simulink model "Corrected_STModel_with_IMM"  (R2019b)
settings: Solver=FixedStepDiscrete  StartTime=0.0  StopTime=6  FixedStep=Ts  RelTol=1e-3  EnableMultiTasking=on
PreLoadFcn:
  | if exist('tl_preloadfcn','file'), tl_preloadfcn(gcs,403); end
PostLoadFcn:
  | if exist('tl_postloadfcn','file'), tl_postloadfcn(gcs,403); end
InitFcn:
  | if exist('tlds_init','file'), tlds_init(gcs); end
StartFcn:
  | if exist('tlds_start','file'), tlds_start(gcs); end
StopFcn:
  | if exist('tlds_stop','file'), tlds_stop(gcs); end
values from neighbouring files (symbols this model uses):
  Bx_ash_f = 11.7    [correctedST_with_behavior_data.m]
  Bx_ash_r = 11.1    [correctedST_with_behavior_data.m]
  Bx_snow_f = 10.2    [correctedST_with_behavior_data.m]
  Bx_snow_r = 9.71    [correctedST_with_behavior_data.m]
  Bx_wash_f = 12    [correctedST_with_behavior_data.m]
  Bx_wash_r = 11.5    [correctedST_with_behavior_data.m]
  By_ash_f = 8.86    [correctedST_with_behavior_data.m]
  By_ash_r = 9.30    (= 9.3)    [correctedST_with_behavior_data.m]
  By_snow_f = 19.1    [correctedST_with_behavior_data.m]
  By_snow_r = 20.0    (= 20)    [correctedST_with_behavior_data.m]
  By_wash_f = 10.7    [correctedST_with_behavior_data.m]
  By_wash_r = 11.3    [correctedST_with_behavior_data.m]
  Cx_ash_f = 1.69    [correctedST_with_behavior_data.m]
  Cx_ash_r = 1.69    [correctedST_with_behavior_data.m]
  Cx_snow_f = 1.96    [correctedST_with_behavior_data.m]
  Cx_snow_r = 1.96    [correctedST_with_behavior_data.m]
  Cx_wash_f = 1.80    (= 1.8)    [correctedST_with_behavior_data.m]
  Cx_wash_r = 1.80    (= 1.8)    [correctedST_with_behavior_data.m]
  Cy_ash_f = 1.19    [correctedST_with_behavior_data.m]
  Cy_ash_r = 1.19    [correctedST_with_behavior_data.m]
  Cy_snow_f = 0.550    (= 0.55)    [correctedST_with_behavior_data.m]
  Cy_snow_r = 0.550    (= 0.55)    [correctedST_with_behavior_data.m]
  Cy_wash_f = 1.07    [correctedST_with_behavior_data.m]
  Cy_wash_r = 1.07    [correctedST_with_behavior_data.m]
  Ex_ash_f = 0.377    [correctedST_with_behavior_data.m]
  Ex_ash_r = 0.362    [correctedST_with_behavior_data.m]
  Ex_snow_f = 0.651    [correctedST_with_behavior_data.m]
  Ex_snow_r = 0.624    [correctedST_with_behavior_data.m]
  Ex_wash_f = 0.313    [correctedST_with_behavior_data.m]
  Ex_wash_r = 0.300    (= 0.3)    [correctedST_with_behavior_data.m]
  Ey_ash_f = -1.21    [correctedST_with_behavior_data.m]
  Ey_ash_r = -1.11    [correctedST_with_behavior_data.m]
  Ey_snow_f = -2.1    [correctedST_with_behavior_data.m]
  Ey_snow_r = -1.93    [correctedST_with_behavior_data.m]
  Ey_wash_f = -2.14    [correctedST_with_behavior_data.m]
  Ey_wash_r = -1.97    [correctedST_with_behavior_data.m]
  g = 9.81    [correctedST_with_behavior_data.m]
  Iw = 4    [correctedST_with_behavior_data.m]
  Iz = 2873    [correctedST_with_behavior_data.m]
  l = l_f+l_r    (= 2.68)    [correctedST_with_behavior_data.m]
  l_f = 1.1    [correctedST_with_behavior_data.m]
  l_r = 1.58    [correctedST_with_behavior_data.m]
  m = 1573    [correctedST_with_behavior_data.m]
  mu_x_ash_f = 1.20    (= 1.2)    [correctedST_with_behavior_data.m]
  mu_x_ash_r = 1.20    (= 1.2)    [correctedST_with_behavior_data.m]
  mu_x_snow_f = 0.407    [correctedST_with_behavior_data.m]
  mu_x_snow_r = 0.409    [correctedST_with_behavior_data.m]
  mu_x_wash_f = 1.06    [correctedST_with_behavior_data.m]
  mu_x_wash_r = 1.07    [correctedST_with_behavior_data.m]
  mu_y_ash_f = 0.935    [correctedST_with_behavior_data.m]
  mu_y_ash_r = 0.961    [correctedST_with_behavior_data.m]
  mu_y_snow_f = 0.383    [correctedST_with_behavior_data.m]
  mu_y_snow_r = 0.394    [correctedST_with_behavior_data.m]
  mu_y_wash_f = 0.885    [correctedST_with_behavior_data.m]
  mu_y_wash_r = 0.911    [correctedST_with_behavior_data.m]
  omega_f0 = Vx0/Rw    (= 33.3333333333)    [correctedST_with_behavior_data.m]
  omega_r0 = Vx0/Rw    (= 33.3333333333)    [correctedST_with_behavior_data.m]
  P_init = 0.0025    [correctedST_with_behavior_data.m]
  psi0 = 0    [correctedST_with_behavior_data.m]
  psi_dot0 = 0    [correctedST_with_behavior_data.m]
  Px0 = 0    [correctedST_with_behavior_data.m]
  Py0 = 0    [correctedST_with_behavior_data.m]
  Re = 0.3    [correctedST_with_behavior_data.m]
  road = 1    [correctedST_with_behavior_data.m]
  Rw = 0.3    [correctedST_with_behavior_data.m]
  Ts = 0.001    [correctedST_with_behavior_data.m]
  Ts_bp = 0.01    [correctedST_with_behavior_data.m]
  Tsmall = 0.001    [correctedST_with_behavior_data.m]
  vx = 10    [correctedST_with_behavior_data.m]
  Vx0 = 10    [correctedST_with_behavior_data.m]
  vy = 0    [correctedST_with_behavior_data.m]
  Vy0 = 0    [correctedST_with_behavior_data.m]
  x = 0    [correctedST_with_behavior_data.m]
  y = 0    [correctedST_with_behavior_data.m]
undefined symbols (not defined in the file or in its folder): DLCTest
libraries: simulink x2
PreSaveFcn:
  | if exist('tl_presavefcn','file'), tl_presavefcn(gcs); end
CloseFcn:
  | if exist('tl_closefcn','file'), tl_closefcn(gcs); end
settings Model: TLRevision=403  ExtModeTrigDuration=10000  Creator=srivats  LastModifiedBy=jasprit
settings SolverCC: PositivePriorityOrder=on  AutoInsertRateTranBlk=on
settings DataIOCC: ReturnWorkspaceOutputs=off
settings DebuggingCC: ArithmeticOperatorsInVariantConditions=warning
settings SFSimCC: SimUseLocalCustomCode=off  CustomCodeUndefinedFunction=UseInterfaceOnly
settings RTWCC: Description=QUARC Win64 Target  SystemTargetFile=quarc_win64.tlc  TemplateMakefile=quarc_default_tmf  RTWUseLocalCustomCode=off
settings STFCustomTargetCC: TargetPreCompLibLocation=C:\PROGRA~3\QUARC\lib\2018a\win64\release  TargetLangStandard=C99 (ISO)  ConcurrentExecutionCompliant=on  GRTInterface=on  SystemTargetFile=quarc_win64.tlc
settings GRTTargetCC: TargetPreCompLibLocation=C:\PROGRA~3\QUARC\lib\2018a\win64\release  ParMdlRefBuildCompliant=off  CompOptLevelCompliant=off  CombineOutputUpdateFcns=off  MatFileLogging=off  CPPClassGenCompliant=off  GRTInterface=on  UseToolchainInfoCompliant=off  ExtMode=on  ExtModeMexFile=quarc_comm

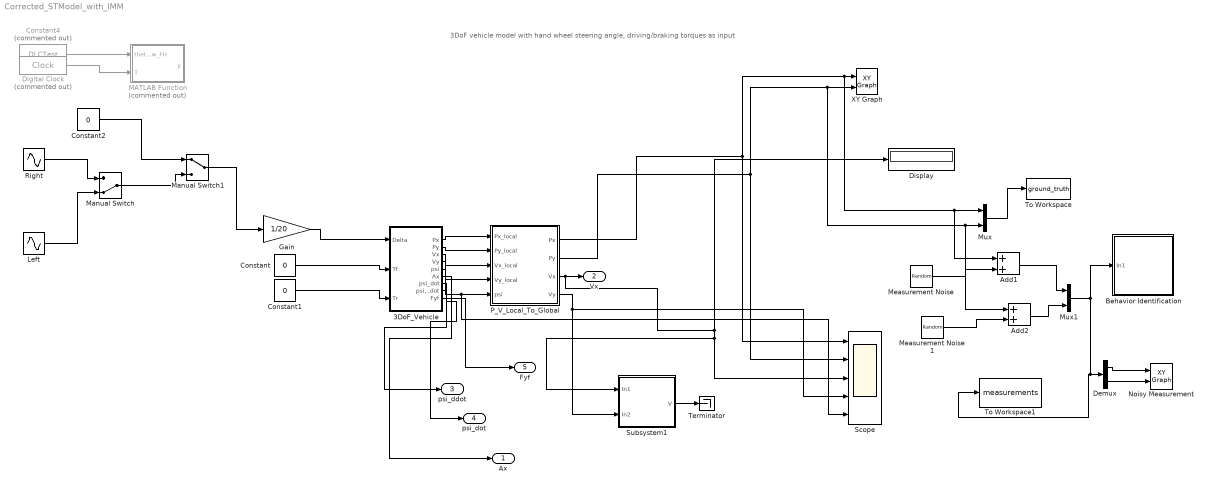
== system Corrected_STModel_with_IMM ==
  note: 3DoF vehicle model with hand wheel steering angle, driving/braking torques as input
  3DoF_Vehicle : Subsystem
  Add1 : Sum
  Add2 : Sum
  Behavior Identification : Subsystem
  Constant : Constant  Value=0
  Constant1 : Constant  Value=0
  Constant2 : Constant  Value=0
  Constant4 : Constant  Commented=on  Value=DLCTest
  Demux : Demux  Outputs=2
  Digital Clock : DigitalClock  Commented=on  SampleTime=0.001
  Display : Display
  Gain : Gain  Gain=1/20
  Left : Sin  Amplitude=0.105  Frequency=2*pi/10  SampleTime=0
  MATLAB Function : MATLAB Function  Commented=on  TreatAsAtomicUnit=on
  Manual Switch : ManualSwitch  CurrentSetting=0
  Manual Switch1 : ManualSwitch
  "Measurement Noise " : RandomNumber  Variance=0.0025
  Measurement Noise 1 : RandomNumber  Variance=0.0025
  Mux : Mux  Inputs=2
  Mux1 : Mux  Inputs=2
  Noisy Measurement : simulink/Sinks/XY Graph  xmin=-10  xmax=100  ymin=-5  ymax=5  st=-1
  P_V_Local_To_Global : Subsystem
  Right : Sin  Amplitude=0.105  Frequency=2*pi/10  Phase=-pi  SampleTime=0
  Scope : Scope  NumInputPorts=5
  Subsystem1 : Subsystem
  Terminator : Terminator
  To Workspace : ToWorkspace  VariableName=ground_truth  SaveFormat=Timeseries  SampleTime=Ts_bp
  To Workspace1 : ToWorkspace  VariableName=measurements  SaveFormat=Timeseries  SampleTime=Ts_bp
  XY Graph : simulink/Sinks/XY Graph  xmin=0  xmax=75  ymin=-4  ymax=4  st=-1
  Ax : Outport  VectorParamsAs1DForOutWhenUnconnected=off
  Vx : Outport  Port=2  VectorParamsAs1DForOutWhenUnconnected=off
  psi_ddot : Outport  Port=3  VectorParamsAs1DForOutWhenUnconnected=off
  psi_dot : Outport  Port=4  VectorParamsAs1DForOutWhenUnconnected=off
  Fyf : Outport  Port=5  VectorParamsAs1DForOutWhenUnconnected=off
  wires:
  P_V_Local_To_Global/4(Vy) -> Scope/4, Subsystem1/2(In2)
  3DoF_Vehicle/5(psi) -> Scope/5, P_V_Local_To_Global/5(psi)
  P_V_Local_To_Global/3(Vx) -> Display/1, Subsystem1/1(In1), Scope/3, Vx/1
  Subsystem1/1(V) -> Terminator/1
  Constant1/1 -> 3DoF_Vehicle/3(Tr)
  3DoF_Vehicle/4(Vy) -> P_V_Local_To_Global/4(Vy_local)
  Constant/1 -> 3DoF_Vehicle/2(Tf)
  3DoF_Vehicle/2(Py) -> P_V_Local_To_Global/2(Py_local)
  3DoF_Vehicle/3(Vx) -> P_V_Local_To_Global/3(Vx_local)
  3DoF_Vehicle/1(Px) -> P_V_Local_To_Global/1(Px_local)
  3DoF_Vehicle/6(Ax) -> Ax/1
  3DoF_Vehicle/8(psi_ddot) -> psi_ddot/1
  3DoF_Vehicle/7(psi_dot) -> psi_dot/1
  3DoF_Vehicle/9(Fyf) -> Fyf/1
  Gain/1 -> 3DoF_Vehicle/1(Delta)
  Constant4/1 -> MATLAB Function/1(theta_sw_FH)
  Digital Clock/1 -> MATLAB Function/2(T)
  Manual Switch/1 -> Manual Switch1/2
  Left/1 -> Manual Switch/2
  Mux/1 -> To Workspace/1
  P_V_Local_To_Global/2(Py) -> Add2/1, Mux/2, XY Graph/2, Scope/2
  P_V_Local_To_Global/1(Px) -> Add1/1, Mux/1, XY Graph/1, Scope/1
  Add1/1 -> Mux1/1
  Demux/1 -> Noisy Measurement/1
  Demux/2 -> Noisy Measurement/2
  Right/1 -> Manual Switch/1
  Constant2/1 -> Manual Switch1/1
  Manual Switch1/1 -> Gain/1
  "Measurement Noise "/1 -> Add1/2
  Measurement Noise 1/1 -> Add2/2
  Add2/1 -> Mux1/2
  Mux1/1 -> Behavior Identification/1(In1), To Workspace1/1, Demux/1

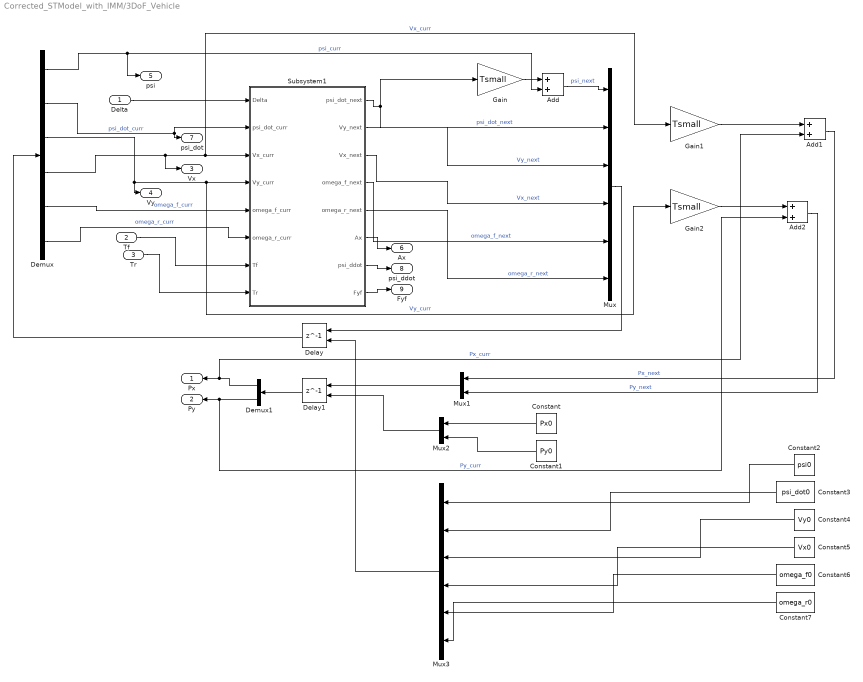
== system Corrected_STModel_with_IMM/3DoF_Vehicle ==
  Delta : Inport
  Tf : Inport  Port=2
  Tr : Inport  Port=3
  Add : Sum
  Add1 : Sum
  Add2 : Sum
  Constant : Constant  Value=Px0
  Constant1 : Constant  Value=Py0
  Constant2 : Constant  Value=psi0
  Constant3 : Constant  Value=psi_dot0
  Constant4 : Constant  Value=Vy0
  Constant5 : Constant  Value=Vx0
  Constant6 : Constant  Value=omega_f0
  Constant7 : Constant  Value=omega_r0
  Delay : Delay  DelayLength=1  InitialConditionSource=Input port  SampleTime=Tsmall
      settings: InputPortMap=u0,p4
  Delay1 : Delay  DelayLength=1  InitialConditionSource=Input port  SampleTime=Tsmall
      settings: InputPortMap=u0,p4
  Demux : Demux  Outputs=6
  Demux1 : Demux  Outputs=2
  Gain : Gain  Gain=Tsmall
  Gain1 : Gain  Gain=Tsmall
  Gain2 : Gain  Gain=Tsmall
  Mux : Mux  Inputs=6
  Mux1 : Mux  Inputs=2
  Mux2 : Mux  Inputs=2
  Mux3 : Mux  Inputs=6
  Subsystem1 : Subsystem
  Px : Outport  VectorParamsAs1DForOutWhenUnconnected=off
  Py : Outport  Port=2  VectorParamsAs1DForOutWhenUnconnected=off
  Vx : Outport  Port=3  VectorParamsAs1DForOutWhenUnconnected=off
  Vy : Outport  Port=4  VectorParamsAs1DForOutWhenUnconnected=off
  psi : Outport  Port=5  VectorParamsAs1DForOutWhenUnconnected=off
  Ax : Outport  Port=6  VectorParamsAs1DForOutWhenUnconnected=off
  psi_dot : Outport  Port=7  VectorParamsAs1DForOutWhenUnconnected=off
  psi_ddot : Outport  Port=8  VectorParamsAs1DForOutWhenUnconnected=off
  Fyf : Outport  Port=9  VectorParamsAs1DForOutWhenUnconnected=off
  wires:
  Demux/1 -> psi/1, Add/2  "psi_curr"
  Delay/1 -> Demux/1
  Demux/6 -> Subsystem1/6(omega_r_curr)  "omega_r_curr"
  Gain/1 -> Add/1
  Delta/1 -> Subsystem1/1(Delta)
  Subsystem1/4(omega_f_next) -> Mux/5  "omega_f_next"
  Subsystem1/1(psi_dot_next) -> Mux/2, Gain/1  "psi_dot_next"
  Add/1 -> Mux/1  "psi_next"
  Tr/1 -> Subsystem1/8(Tr)
  Tf/1 -> Subsystem1/7(Tf)
  Subsystem1/3(Vx_next) -> Mux/4  "Vx_next"
  Demux/2 -> psi_dot/1, Subsystem1/2(psi_dot_curr)  "psi_dot_curr"
  Mux/1 -> Delay/1
  Demux/4 -> Vx/1, Gain1/1, Subsystem1/3(Vx_curr)  "Vx_curr"
  Demux/3 -> Gain2/1, Subsystem1/4(Vy_curr), Vy/1  "Vy_curr"
  Demux/5 -> Subsystem1/5(omega_f_curr)  "omega_f_curr"
  Subsystem1/2(Vy_next) -> Mux/3  "Vy_next"
  Subsystem1/5(omega_r_next) -> Mux/6  "omega_r_next"
  Gain1/1 -> Add1/1
  Gain2/1 -> Add2/1
  Mux1/1 -> Delay1/1
  Add1/1 -> Mux1/1  "Px_next"
  Add2/1 -> Mux1/2  "Py_next"
  Mux2/1 -> Delay1/2
  Constant/1 -> Mux2/1
  Constant1/1 -> Mux2/2
  Delay1/1 -> Demux1/1
  Demux1/1 -> Add1/2, Px/1  "Px_curr"
  Demux1/2 -> Add2/2, Py/1  "Py_curr"
  Constant7/1 -> Mux3/6
  Constant6/1 -> Mux3/5
  Constant3/1 -> Mux3/2
  Constant5/1 -> Mux3/4
  Constant4/1 -> Mux3/3
  Constant2/1 -> Mux3/1
  Mux3/1 -> Delay/2
  Subsystem1/6(Ax) -> Ax/1
  Subsystem1/7(psi_ddot) -> psi_ddot/1
  Subsystem1/8(Fyf) -> Fyf/1

== system Corrected_STModel_with_IMM/Behavior Identification ==
  In1 : Inport  SampleTime=Ts_bp
  Constant : Constant  Value=0
  MATLAB Function3 : MATLAB Function  TreatAsAtomicUnit=on
  P_init : Constant  Value=P_init * eye(4)  SampleTime=-1
  To Workspace2 : ToWorkspace  VariableName=imm_comb_estimate  SaveFormat=Timeseries  SampleTime=-1
  combined Estimate : Scope
  estimates : Scope
  likelihoods : Scope
  prenormalized Wts : Scope
  weights : Scope
  x_init : Constant  Value=[x vx y vy]'
  wires:
  Constant/1 -> MATLAB Function3/2(u)
  MATLAB Function3/2(weights) -> weights/1
  MATLAB Function3/1(prenormalizedWts) -> prenormalized Wts/1
  MATLAB Function3/4(estimates) -> estimates/1
  x_init/1 -> MATLAB Function3/3(X)
  P_init/1 -> MATLAB Function3/4(P)
  MATLAB Function3/3(likelihood) -> likelihoods/1
  MATLAB Function3/5(comb_x) -> To Workspace2/1, combined Estimate/1
  In1/1 -> MATLAB Function3/1(y_tilde)

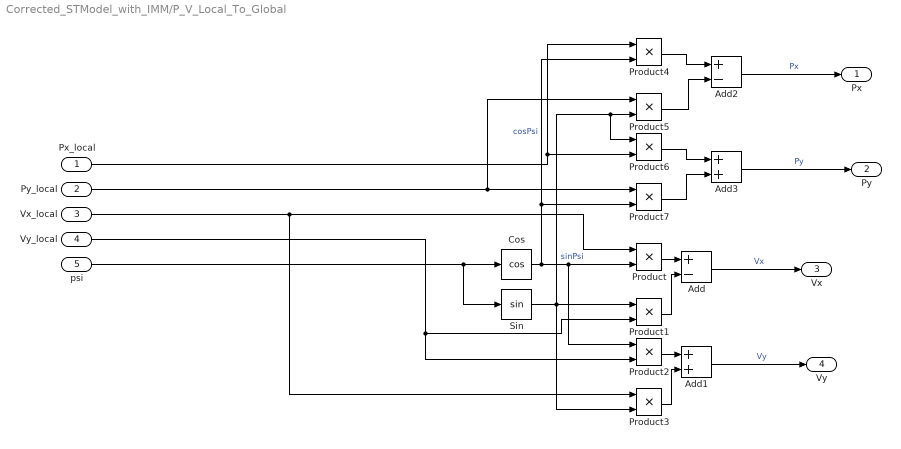
== system Corrected_STModel_with_IMM/P_V_Local_To_Global ==
  Px_local : Inport  OutDataTypeStr=double  SampleTime=Ts
  Py_local : Inport  Port=2  OutDataTypeStr=double  SampleTime=Ts
  Vx_local : Inport  Port=3  OutDataTypeStr=double  SampleTime=Ts
  Vy_local : Inport  Port=4  OutDataTypeStr=double  SampleTime=Ts
  psi : Inport  Port=5  OutDataTypeStr=double  SampleTime=Ts
  Add : Sum  Inputs=+-
  Add1 : Sum
  Add2 : Sum  Inputs=+-
  Add3 : Sum
  Cos : Trigonometry  Operator=cos
  Product{,1..7} (8 alike) : Product
  Sin : Trigonometry
  Px : Outport  OutDataTypeStr=double  SampleTime=Ts  VectorParamsAs1DForOutWhenUnconnected=off
  Py : Outport  Port=2  OutDataTypeStr=double  SampleTime=Ts  VectorParamsAs1DForOutWhenUnconnected=off
  Vx : Outport  Port=3  OutDataTypeStr=double  SampleTime=Ts  VectorParamsAs1DForOutWhenUnconnected=off
  Vy : Outport  Port=4  OutDataTypeStr=double  SampleTime=Ts  VectorParamsAs1DForOutWhenUnconnected=off
  wires:
  Px_local/1 -> Product4/1, Product6/2
  Py_local/1 -> Product7/1, Product5/1
  Vx_local/1 -> Product3/1, Product/1
  Product5/1 -> Add2/2
  Product4/1 -> Add2/1
  Add2/1 -> Px/1  "Px"
  Product7/1 -> Add3/2
  Sin/1 -> Product6/1, Product5/2, Product3/2, Product1/1  "sinPsi"
  Vy_local/1 -> Product1/2, Product2/2
  psi/1 -> Sin/1, Cos/1
  Cos/1 -> Product7/2, Product4/2, Product2/1, Product/2  "cosPsi"
  Add3/1 -> Py/1  "Py"
  Product2/1 -> Add1/1
  Product1/1 -> Add/2
  Add/1 -> Vx/1  "Vx"
  Add1/1 -> Vy/1  "Vy"
  Product6/1 -> Add3/1
  Product3/1 -> Add1/2
  Product/1 -> Add/1

== system Corrected_STModel_with_IMM/Subsystem1 ==
  In1 : Inport
  In2 : Inport  Port=2
  Add : Sum
  Sqrt : Sqrt  SaturateOnIntegerOverflow=on
  Square : Math  Operator=square  SaturateOnIntegerOverflow=on
  Square1 : Math  Operator=square  SaturateOnIntegerOverflow=on
  V : Outport  VectorParamsAs1DForOutWhenUnconnected=off
  wires:
  Square1/1 -> Add/2
  In1/1 -> Square/1
  Add/1 -> Sqrt/1
  Square/1 -> Add/1
  Sqrt/1 -> V/1  "V"
  In2/1 -> Square1/1

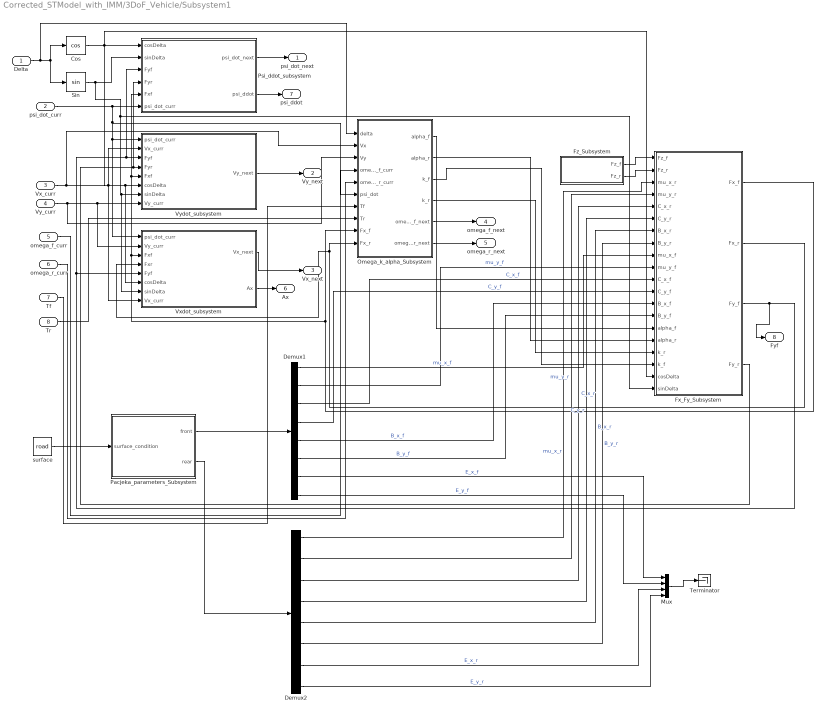
== system Corrected_STModel_with_IMM/3DoF_Vehicle/Subsystem1 ==
  Delta : Inport
  psi_dot_curr : Inport  Port=2
  Vx_curr : Inport  Port=3
  Vy_curr : Inport  Port=4
  omega_f_curr : Inport  Port=5
  omega_r_curr : Inport  Port=6
  Tf : Inport  Port=7
  Tr : Inport  Port=8
  Cos : Trigonometry  Operator=cos
  Demux1 : Demux  Outputs=8
  Demux2 : Demux  Outputs=8
  Fx_Fy_Subsystem : Subsystem
  Fz_Subsystem : Subsystem
  Mux : Mux
  Omega_k_alpha_Subsystem : Subsystem
  Pacjeka_parameters_Subsystem : Subsystem
  Psi_ddot_subsystem : Subsystem
  Sin : Trigonometry
  Terminator : Terminator
  Vxdot_subsystem : Subsystem
  Vydot_subsystem : Subsystem
  surface : Constant  Value=road
  psi_dot_next : Outport  VectorParamsAs1DForOutWhenUnconnected=off
  Vy_next : Outport  Port=2  VectorParamsAs1DForOutWhenUnconnected=off
  Vx_next : Outport  Port=3  VectorParamsAs1DForOutWhenUnconnected=off
  omega_f_next : Outport  Port=4  VectorParamsAs1DForOutWhenUnconnected=off
  omega_r_next : Outport  Port=5  VectorParamsAs1DForOutWhenUnconnected=off
  Ax : Outport  Port=6  VectorParamsAs1DForOutWhenUnconnected=off
  psi_ddot : Outport  Port=7  VectorParamsAs1DForOutWhenUnconnected=off
  Fyf : Outport  Port=8  VectorParamsAs1DForOutWhenUnconnected=off
  wires:
  Omega_k_alpha_Subsystem/4(k_r) -> Fx_Fy_Subsystem/17(k_r)
  Fx_Fy_Subsystem/2(Fx_r) -> Vxdot_subsystem/4(Fxr), Omega_k_alpha_Subsystem/10(Fx_r)
  Fx_Fy_Subsystem/1(Fx_f) -> Omega_k_alpha_Subsystem/9(Fx_f), Vxdot_subsystem/3(Fxf), Psi_ddot_subsystem/5(Fxf), Vydot_subsystem/5(Fxf)
  Omega_k_alpha_Subsystem/3(k_f) -> Fx_Fy_Subsystem/18(k_f)
  Sin/1 -> Fx_Fy_Subsystem/20(sinDelta), Vxdot_subsystem/7(sinDelta), Vydot_subsystem/7(sinDelta), Psi_ddot_subsystem/2(sinDelta)
  Vydot_subsystem/1(Vy_next) -> Vy_next/1
  Fx_Fy_Subsystem/3(Fy_f) -> Fyf/1, Psi_ddot_subsystem/3(Fyf), Vydot_subsystem/3(Fyf), Vxdot_subsystem/5(Fyf)
  psi_dot_curr/1 -> Omega_k_alpha_Subsystem/6(psi_dot), Vydot_subsystem/1(psi_dot_curr), Vxdot_subsystem/1(psi_dot_curr), Psi_ddot_subsystem/6(psi_dot_curr)
  Fx_Fy_Subsystem/4(Fy_r) -> Psi_ddot_subsystem/4(Fyr), Vydot_subsystem/4(Fyr)
  Cos/1 -> Fx_Fy_Subsystem/19(cosDelta), Vxdot_subsystem/6(cosDelta), Vydot_subsystem/6(cosDelta), Psi_ddot_subsystem/1(cosDelta)
  Tf/1 -> Omega_k_alpha_Subsystem/7(Tf)
  omega_f_curr/1 -> Omega_k_alpha_Subsystem/4(omega_f_curr)
  Vy_curr/1 -> Omega_k_alpha_Subsystem/3(Vy), Vxdot_subsystem/2(Vy_curr), Vydot_subsystem/8(Vy_curr)
  Pacjeka_parameters_Subsystem/1(front) -> Demux1/1
  Omega_k_alpha_Subsystem/6(omega_r_next) -> omega_r_next/1
  Delta/1 -> Omega_k_alpha_Subsystem/1(delta), Sin/1, Cos/1
  Vx_curr/1 -> Omega_k_alpha_Subsystem/2(Vx), Vydot_subsystem/2(Vx_curr), Vxdot_subsystem/8(Vx_curr)
  Demux1/1 -> Fx_Fy_Subsystem/9(mu_x_f)  "mu_x_f"
  Vxdot_subsystem/1(Vx_next) -> Vx_next/1
  Omega_k_alpha_Subsystem/5(omega_f_next) -> omega_f_next/1
  Demux2/4 -> Fx_Fy_Subsystem/6(C_y_r)  "C_y_r"
  Fz_Subsystem/1(Fz_f) -> Fx_Fy_Subsystem/1(Fz_f)
  Tr/1 -> Omega_k_alpha_Subsystem/8(Tr)
  omega_r_curr/1 -> Omega_k_alpha_Subsystem/5(omega_r_curr)
  surface/1 -> Pacjeka_parameters_Subsystem/1(surface_condition)
  Pacjeka_parameters_Subsystem/2(rear) -> Demux2/1
  Fz_Subsystem/2(Fz_r) -> Fx_Fy_Subsystem/2(Fz_r)
  Demux1/6 -> Fx_Fy_Subsystem/14(B_y_f)  "B_y_f"
  Demux2/6 -> Fx_Fy_Subsystem/8(B_y_r)  "B_y_r"
  Demux2/2 -> Fx_Fy_Subsystem/4(mu_y_r)  "mu_y_r"
  Demux2/5 -> Fx_Fy_Subsystem/7(B_x_r)  "B_x_r"
  Psi_ddot_subsystem/1(psi_dot_next) -> psi_dot_next/1
  Demux2/1 -> Fx_Fy_Subsystem/3(mu_x_r)  "mu_x_r"
  Demux1/3 -> Fx_Fy_Subsystem/11(C_x_f)  "C_x_f"
  Demux1/4 -> Fx_Fy_Subsystem/12(C_y_f)  "C_y_f"
  Demux1/2 -> Fx_Fy_Subsystem/10(mu_y_f)  "mu_y_f"
  Demux1/5 -> Fx_Fy_Subsystem/13(B_x_f)  "B_x_f"
  Demux2/3 -> Fx_Fy_Subsystem/5(C_x_r)  "C_x_r"
  Vxdot_subsystem/2(Ax) -> Ax/1
  Psi_ddot_subsystem/2(psi_ddot) -> psi_ddot/1
  Omega_k_alpha_Subsystem/1(alpha_f) -> Fx_Fy_Subsystem/15(alpha_f)
  Omega_k_alpha_Subsystem/2(alpha_r) -> Fx_Fy_Subsystem/16(alpha_r)
  Demux1/8 -> Mux/2  "E_y_f"
  Demux1/7 -> Mux/1  "E_x_f"
  Demux2/7 -> Mux/3  "E_x_r"
  Demux2/8 -> Mux/4  "E_y_r"
  Mux/1 -> Terminator/1

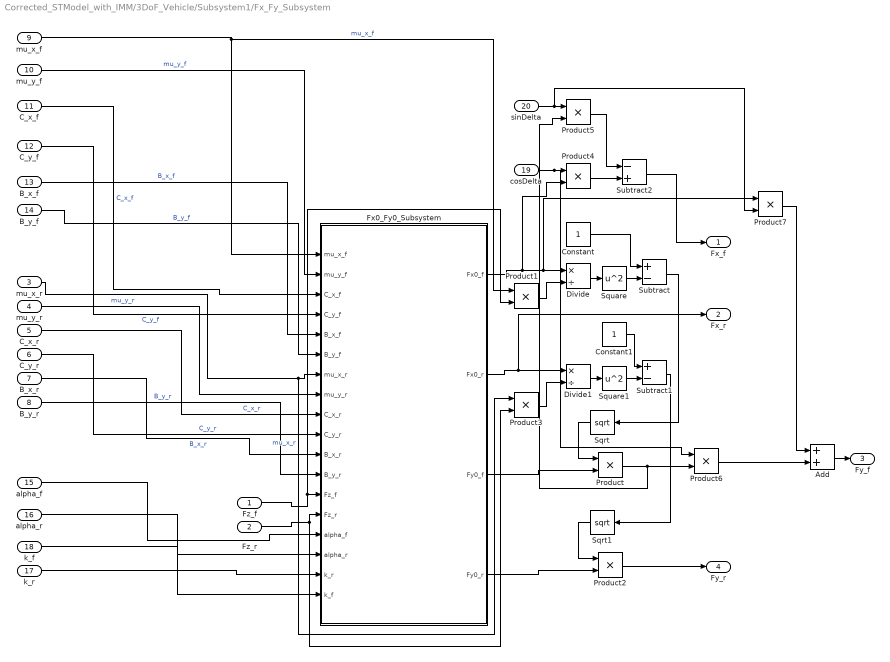
== system Corrected_STModel_with_IMM/3DoF_Vehicle/Subsystem1/Fx_Fy_Subsystem ==
  Fz_f : Inport
  Fz_r : Inport  Port=2
  mu_x_r : Inport  Port=3
  mu_y_r : Inport  Port=4
  C_x_r : Inport  Port=5
  C_y_r : Inport  Port=6
  B_x_r : Inport  Port=7
  B_y_r : Inport  Port=8
  mu_x_f : Inport  Port=9
  mu_y_f : Inport  Port=10
  C_x_f : Inport  Port=11
  C_y_f : Inport  Port=12
  B_x_f : Inport  Port=13
  B_y_f : Inport  Port=14
  alpha_f : Inport  Port=15
  alpha_r : Inport  Port=16
  k_r : Inport  Port=17
  k_f : Inport  Port=18
  cosDelta : Inport  Port=19
  sinDelta : Inport  Port=20
  Add : Sum
  Constant : Constant
  Constant1 : Constant
  Divide : Product  Inputs=*/
  Divide1 : Product  Inputs=*/
  Fx0_Fy0_Subsystem : Subsystem
  Product{,1..7} (8 alike) : Product
  Sqrt : Sqrt  SaturateOnIntegerOverflow=on
  Sqrt1 : Sqrt  SaturateOnIntegerOverflow=on
  Square : Math  Operator=square  SaturateOnIntegerOverflow=on
  Square1 : Math  Operator=square  SaturateOnIntegerOverflow=on
  Subtract : Sum  Inputs=+-
  Subtract1 : Sum  Inputs=+-
  Subtract2 : Sum  Inputs=-+
  Fx_f : Outport  VectorParamsAs1DForOutWhenUnconnected=off
  Fx_r : Outport  Port=2  VectorParamsAs1DForOutWhenUnconnected=off
  Fy_f : Outport  Port=3  VectorParamsAs1DForOutWhenUnconnected=off
  Fy_r : Outport  Port=4  VectorParamsAs1DForOutWhenUnconnected=off
  wires:
  B_x_r/1 -> Fx0_Fy0_Subsystem/11(B_x_r)  "B_x_r"
  mu_y_r/1 -> Fx0_Fy0_Subsystem/8(mu_y_r)  "mu_y_r"
  C_x_r/1 -> Fx0_Fy0_Subsystem/9(C_x_r)  "C_x_r"
  mu_x_r/1 -> Fx0_Fy0_Subsystem/7(mu_x_r), Product3/1  "mu_x_r"
  C_y_r/1 -> Fx0_Fy0_Subsystem/10(C_y_r)  "C_y_r"
  B_y_r/1 -> Fx0_Fy0_Subsystem/12(B_y_r)  "B_y_r"
  B_x_f/1 -> Fx0_Fy0_Subsystem/5(B_x_f)  "B_x_f"
  mu_y_f/1 -> Fx0_Fy0_Subsystem/2(mu_y_f)  "mu_y_f"
  C_x_f/1 -> Fx0_Fy0_Subsystem/3(C_x_f)  "C_x_f"
  mu_x_f/1 -> Product1/1, Fx0_Fy0_Subsystem/1(mu_x_f)  "mu_x_f"
  C_y_f/1 -> Fx0_Fy0_Subsystem/4(C_y_f)  "C_y_f"
  B_y_f/1 -> Fx0_Fy0_Subsystem/6(B_y_f)  "B_y_f"
  Fz_f/1 -> Product1/2, Fx0_Fy0_Subsystem/13(Fz_f)
  Fz_r/1 -> Product3/2, Fx0_Fy0_Subsystem/14(Fz_r)
  alpha_f/1 -> Fx0_Fy0_Subsystem/15(alpha_f)
  alpha_r/1 -> Fx0_Fy0_Subsystem/16(alpha_r)
  k_f/1 -> Fx0_Fy0_Subsystem/18(k_f)
  k_r/1 -> Fx0_Fy0_Subsystem/17(k_r)
  Constant/1 -> Subtract/1
  Fx0_Fy0_Subsystem/1(Fx0_f) -> Product4/2, Product7/1, Divide/1
  Product1/1 -> Divide/2
  Divide/1 -> Square/1
  Subtract/1 -> Sqrt/1
  Square/1 -> Subtract/2
  Sqrt/1 -> Product/1
  Product/1 -> Product6/2, Product5/2
  Product2/1 -> Fy_r/1
  Fx0_Fy0_Subsystem/4(Fy0_r) -> Product2/2
  Sqrt1/1 -> Product2/1
  Divide1/1 -> Square1/1
  Square1/1 -> Subtract1/2
  Product3/1 -> Divide1/2
  Fx0_Fy0_Subsystem/2(Fx0_r) -> Fx_r/1, Divide1/1
  Constant1/1 -> Subtract1/1
  Subtract1/1 -> Sqrt1/1
  cosDelta/1 -> Product6/1, Product4/1
  Product4/1 -> Subtract2/2
  sinDelta/1 -> Product7/2, Product5/1
  Fx0_Fy0_Subsystem/3(Fy0_f) -> Product/2
  Product5/1 -> Subtract2/1
  Subtract2/1 -> Fx_f/1
  Product7/1 -> Add/1
  Product6/1 -> Add/2
  Add/1 -> Fy_f/1

== system Corrected_STModel_with_IMM/3DoF_Vehicle/Subsystem1/Fz_Subsystem ==
  Constant : Constant  Value=(m*g*l_f)/l
  Constant1 : Constant  Value=(m*g*l_r)/l
  Fz_f : Outport  VectorParamsAs1DForOutWhenUnconnected=off
  Fz_r : Outport  Port=2  VectorParamsAs1DForOutWhenUnconnected=off
  wires:
  Constant/1 -> Fz_r/1
  Constant1/1 -> Fz_f/1

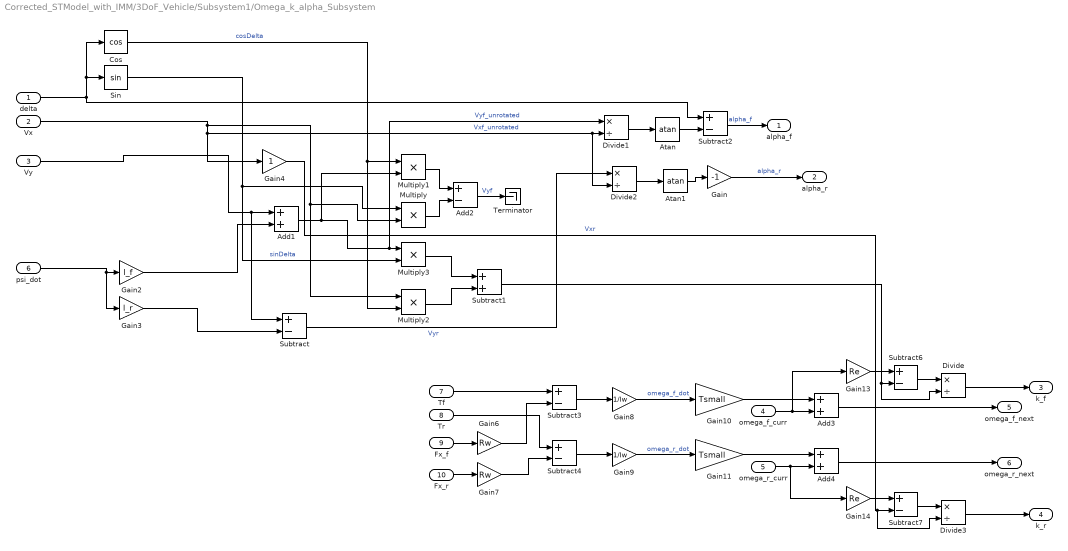
== system Corrected_STModel_with_IMM/3DoF_Vehicle/Subsystem1/Omega_k_alpha_Subsystem ==
  delta : Inport
  Vx : Inport  Port=2
  Vy : Inport  Port=3
  omega_f_curr : Inport  Port=4
  omega_r_curr : Inport  Port=5
  psi_dot : Inport  Port=6
  Tf : Inport  Port=7
  Tr : Inport  Port=8
  Fx_f : Inport  Port=9
  Fx_r : Inport  Port=10
  Add1 : Sum
  Add2 : Sum  Inputs=+-
  Add3 : Sum
  Add4 : Sum
  Atan : Trigonometry  Operator=atan
  Atan1 : Trigonometry  Operator=atan
  Cos : Trigonometry  Operator=cos
  Divide{,1..3} (4 alike) : Product  Inputs=*/
  Gain : Gain  Gain=-1
  Gain10 : Gain  Gain=Tsmall
  Gain11 : Gain  Gain=Tsmall
  Gain13 : Gain  Gain=Re
  Gain14 : Gain  Gain=Re
  Gain2 : Gain  Gain=l_f
  Gain3 : Gain  Gain=l_r
  Gain4 : Gain
  Gain6 : Gain  Gain=Rw
  Gain7 : Gain  Gain=Rw
  Gain8 : Gain  Gain=1/Iw
  Gain9 : Gain  Gain=1/Iw
  Multiply{,1..3} (4 alike) : Product
  Sin : Trigonometry
  Subtract{,2..4,6..7} (6 alike) : Sum  Inputs=+-
  Subtract1 : Sum
  Terminator : Terminator
  alpha_f : Outport  VectorParamsAs1DForOutWhenUnconnected=off
  alpha_r : Outport  Port=2  VectorParamsAs1DForOutWhenUnconnected=off
  k_f : Outport  Port=3  VectorParamsAs1DForOutWhenUnconnected=off
  k_r : Outport  Port=4  VectorParamsAs1DForOutWhenUnconnected=off
  omega_f_next : Outport  Port=5  VectorParamsAs1DForOutWhenUnconnected=off
  omega_r_next : Outport  Port=6  VectorParamsAs1DForOutWhenUnconnected=off
  wires:
  Fx_f/1 -> Gain6/1
  Fx_r/1 -> Gain7/1
  Tf/1 -> Subtract3/1
  Gain6/1 -> Subtract3/2
  Tr/1 -> Subtract4/1
  Gain7/1 -> Subtract4/2
  Subtract3/1 -> Gain8/1
  Subtract4/1 -> Gain9/1
  Gain8/1 -> Gain10/1  "omega_f_dot"
  Gain9/1 -> Gain11/1  "omega_r_dot"
  Gain10/1 -> Add3/1
  Gain11/1 -> Add4/1
  Add3/1 -> omega_f_next/1
  Add4/1 -> omega_r_next/1
  omega_f_curr/1 -> Gain13/1, Add3/2
  omega_r_curr/1 -> Gain14/1, Add4/2
  psi_dot/1 -> Gain3/1, Gain2/1
  Gain2/1 -> Add1/2
  Vy/1 -> Subtract/1, Add1/1
  Add1/1 -> Multiply1/2, Divide1/1, Multiply3/1  "Vyf_unrotated"
  Gain3/1 -> Subtract/2
  Vx/1 -> Gain4/1, Divide2/2, Divide1/2, Multiply/2, Multiply2/1  "Vxf_unrotated"
  Gain4/1 -> Divide3/2, Subtract7/2  "Vxr"
  delta/1 -> Cos/1, Sin/1, Subtract2/1
  Cos/1 -> Multiply2/2, Multiply1/1  "cosDelta"
  Multiply1/1 -> Add2/1
  Multiply/1 -> Add2/2
  Multiply3/1 -> Subtract1/1
  Multiply2/1 -> Subtract1/2
  Gain13/1 -> Subtract6/1
  Subtract6/1 -> Divide/1
  Divide/1 -> k_f/1
  Gain14/1 -> Subtract7/1
  Subtract7/1 -> Divide3/1
  Divide3/1 -> k_r/1
  Sin/1 -> Multiply/1, Multiply3/2  "sinDelta"
  Subtract1/1 -> Divide/2, Subtract6/2
  Subtract/1 -> Divide2/1  "Vyr"
  Divide1/1 -> Atan/1
  Atan/1 -> Subtract2/2
  Subtract2/1 -> alpha_f/1  "alpha_f"
  Divide2/1 -> Atan1/1
  Atan1/1 -> Gain/1
  Gain/1 -> alpha_r/1  "alpha_r"
  Add2/1 -> Terminator/1  "Vyf"

== system Corrected_STModel_with_IMM/3DoF_Vehicle/Subsystem1/Pacjeka_parameters_Subsystem ==
  surface_condition : Inport  OutDataTypeStr=double  SampleTime=Ts
  Ashphalt_condition_subsystem : Subsystem  TreatAsAtomicUnit=on
  Demux : Demux  Outputs=2
  Ice_condition_subsystem : Subsystem  TreatAsAtomicUnit=on
  Merge : Merge  Inputs=4
  Snow_condition_subsystem : Subsystem  TreatAsAtomicUnit=on
  Switch Case : SwitchCase  CaseConditions={1,2,3,4}  ShowDefaultCase=off
  WetAshphalt_condition_subsystem : Subsystem  TreatAsAtomicUnit=on
  front : Outport  OutDataTypeStr=double  SampleTime=Ts  VectorParamsAs1DForOutWhenUnconnected=off
  rear : Outport  Port=2  OutDataTypeStr=double  SampleTime=Ts  VectorParamsAs1DForOutWhenUnconnected=off
  wires:
  Demux/2 -> rear/1  "rear"
  Merge/1 -> Demux/1
  Switch Case/1 -> Ashphalt_condition_subsystem/Action
  Switch Case/3 -> Snow_condition_subsystem/Action
  Demux/1 -> front/1  "front"
  surface_condition/1 -> Switch Case/1
  Ashphalt_condition_subsystem/1(Out1) -> Merge/1
  Switch Case/2 -> WetAshphalt_condition_subsystem/Action
  WetAshphalt_condition_subsystem/1(Out1) -> Merge/2
  Snow_condition_subsystem/1(Out1) -> Merge/3
  Ice_condition_subsystem/1(Out1) -> Merge/4
  Switch Case/4 -> Ice_condition_subsystem/Action

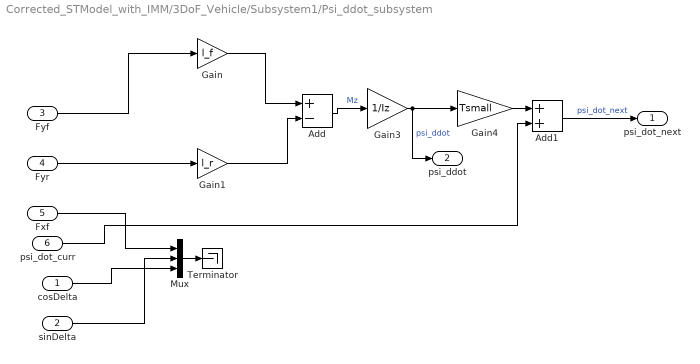
== system Corrected_STModel_with_IMM/3DoF_Vehicle/Subsystem1/Psi_ddot_subsystem ==
  cosDelta : Inport
  sinDelta : Inport  Port=2
  Fyf : Inport  Port=3
  Fyr : Inport  Port=4
  Fxf : Inport  Port=5
  psi_dot_curr : Inport  Port=6
  Add : Sum  Inputs=+-
  Add1 : Sum
  Gain : Gain  Gain=l_f
  Gain1 : Gain  Gain=l_r
  Gain3 : Gain  Gain=1/Iz
  Gain4 : Gain  Gain=Tsmall
  Mux : Mux  Inputs=3
  Terminator : Terminator
  psi_dot_next : Outport  VectorParamsAs1DForOutWhenUnconnected=off
  psi_ddot : Outport  Port=2  VectorParamsAs1DForOutWhenUnconnected=off
  wires:
  Gain/1 -> Add/1
  Gain1/1 -> Add/2
  Add/1 -> Gain3/1  "Mz"
  Gain3/1 -> psi_ddot/1, Gain4/1  "psi_ddot"
  Gain4/1 -> Add1/1
  Add1/1 -> psi_dot_next/1  "psi_dot_next"
  Fyf/1 -> Gain/1
  Fyr/1 -> Gain1/1
  psi_dot_curr/1 -> Add1/2
  cosDelta/1 -> Mux/3
  Fxf/1 -> Mux/1
  sinDelta/1 -> Mux/2
  Mux/1 -> Terminator/1

== system Corrected_STModel_with_IMM/3DoF_Vehicle/Subsystem1/Vxdot_subsystem ==
  psi_dot_curr : Inport
  Vy_curr : Inport  Port=2
  Fxf : Inport  Port=3
  Fxr : Inport  Port=4
  Fyf : Inport  Port=5
  cosDelta : Inport  Port=6
  sinDelta : Inport  Port=7
  Vx_curr : Inport  Port=8
  Add : Sum
  Fy_subsystem : Subsystem
  Gain : Gain  Gain=1/m
  Gain1 : Gain  Gain=Ts
  Multiply : Product
  Subtract : Sum
  Vx_next : Outport  VectorParamsAs1DForOutWhenUnconnected=off
  Ax : Outport  Port=2  VectorParamsAs1DForOutWhenUnconnected=off
  wires:
  sinDelta/1 -> Fy_subsystem/5(sinDelta)
  cosDelta/1 -> Fy_subsystem/4(cosDelta)
  Fyf/1 -> Fy_subsystem/3(Fxr)
  Fxr/1 -> Fy_subsystem/2(Fxf)
  Fxf/1 -> Fy_subsystem/1(Fyf)
  Fy_subsystem/1(Fx) -> Gain/1
  Gain/1 -> Subtract/2
  psi_dot_curr/1 -> Multiply/1
  Vy_curr/1 -> Multiply/2
  Multiply/1 -> Subtract/1
  Subtract/1 -> Ax/1, Gain1/1
  Gain1/1 -> Add/1
  Vx_curr/1 -> Add/2
  Add/1 -> Vx_next/1  "Vx_next"

== system Corrected_STModel_with_IMM/3DoF_Vehicle/Subsystem1/Vydot_subsystem ==
  psi_dot_curr : Inport
  Vx_curr : Inport  Port=2
  Fyf : Inport  Port=3
  Fyr : Inport  Port=4
  Fxf : Inport  Port=5
  cosDelta : Inport  Port=6
  sinDelta : Inport  Port=7
  Vy_curr : Inport  Port=8
  Add : Sum
  Fy_subsystem : Subsystem
  Gain : Gain  Gain=1/m
  Gain1 : Gain  Gain=Ts
  Multiply : Product
  Subtract : Sum  Inputs=-+
  Vy_next : Outport  VectorParamsAs1DForOutWhenUnconnected=off
  wires:
  sinDelta/1 -> Fy_subsystem/5(sinDelta)
  cosDelta/1 -> Fy_subsystem/4(cosDelta)
  Fxf/1 -> Fy_subsystem/3(Fxf)
  Fyr/1 -> Fy_subsystem/2(Fyr)
  Fyf/1 -> Fy_subsystem/1(Fyf)
  Fy_subsystem/1(Fy) -> Gain/1
  Gain/1 -> Subtract/2
  psi_dot_curr/1 -> Multiply/1
  Vx_curr/1 -> Multiply/2
  Multiply/1 -> Subtract/1
  Subtract/1 -> Gain1/1
  Gain1/1 -> Add/1
  Vy_curr/1 -> Add/2
  Add/1 -> Vy_next/1  "Vy_next"

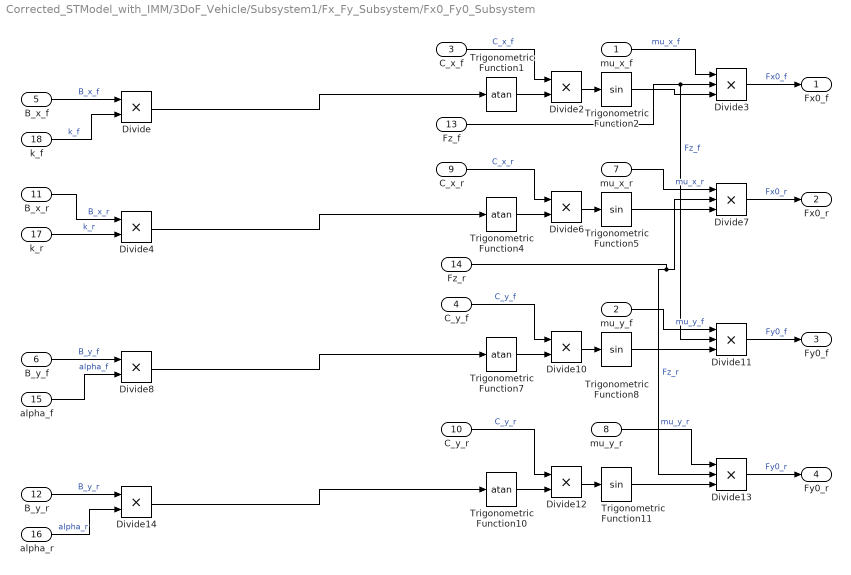
== system Corrected_STModel_with_IMM/3DoF_Vehicle/Subsystem1/Fx_Fy_Subsystem/Fx0_Fy0_Subsystem ==
  mu_x_f : Inport
  mu_y_f : Inport  Port=2
  C_x_f : Inport  Port=3
  C_y_f : Inport  Port=4
  B_x_f : Inport  Port=5
  B_y_f : Inport  Port=6
  mu_x_r : Inport  Port=7
  mu_y_r : Inport  Port=8
  C_x_r : Inport  Port=9
  C_y_r : Inport  Port=10
  B_x_r : Inport  Port=11
  B_y_r : Inport  Port=12
  Fz_f : Inport  Port=13
  Fz_r : Inport  Port=14
  alpha_f : Inport  Port=15
  alpha_r : Inport  Port=16
  k_r : Inport  Port=17
  k_f : Inport  Port=18
  Divide{,2,4,6,8,10,12,14} (8 alike) : Product  Inputs=**
  Divide{3,7,11,13} (4 alike) : Product  Inputs=***
  Trigonometric Function{1,4,7,10} (4 alike) : Trigonometry  Operator=atan
  Trigonometric Function{2,5,8,11} (4 alike) : Trigonometry
  Fx0_f : Outport  VectorParamsAs1DForOutWhenUnconnected=off
  Fx0_r : Outport  Port=2  VectorParamsAs1DForOutWhenUnconnected=off
  Fy0_f : Outport  Port=3  VectorParamsAs1DForOutWhenUnconnected=off
  Fy0_r : Outport  Port=4  VectorParamsAs1DForOutWhenUnconnected=off
  wires:
  B_x_f/1 -> Divide/1  "B_x_f"
  C_x_f/1 -> Divide2/1  "C_x_f"
  mu_x_f/1 -> Divide3/1  "mu_x_f"
  mu_y_f/1 -> Divide11/1  "mu_y_f"
  B_y_f/1 -> Divide8/1  "B_y_f"
  C_y_f/1 -> Divide10/1  "C_y_f"
  B_y_r/1 -> Divide14/1  "B_y_r"
  mu_x_r/1 -> Divide7/1  "mu_x_r"
  B_x_r/1 -> Divide4/1  "B_x_r"
  mu_y_r/1 -> Divide13/1  "mu_y_r"
  C_y_r/1 -> Divide12/1  "C_y_r"
  C_x_r/1 -> Divide6/1  "C_x_r"
  Trigonometric Function2/1 -> Divide3/3
  Divide3/1 -> Fx0_f/1  "Fx0_f"
  Trigonometric Function5/1 -> Divide7/3
  Divide4/1 -> Trigonometric Function4/1
  Divide2/1 -> Trigonometric Function2/1
  Divide/1 -> Trigonometric Function1/1
  Trigonometric Function4/1 -> Divide6/2
  Divide7/1 -> Fx0_r/1  "Fx0_r"
  Divide6/1 -> Trigonometric Function5/1
  Trigonometric Function1/1 -> Divide2/2
  alpha_f/1 -> Divide8/2  "alpha_f"
  alpha_r/1 -> Divide14/2  "alpha_r"
  k_f/1 -> Divide/2  "k_f"
  k_r/1 -> Divide4/2  "k_r"
  Trigonometric Function7/1 -> Divide10/2
  Divide10/1 -> Trigonometric Function8/1
  Fz_f/1 -> Divide11/2, Divide3/2  "Fz_f"
  Divide8/1 -> Trigonometric Function7/1
  Trigonometric Function8/1 -> Divide11/3
  Divide11/1 -> Fy0_f/1  "Fy0_f"
  Divide13/1 -> Fy0_r/1  "Fy0_r"
  Fz_r/1 -> Divide13/2, Divide7/2  "Fz_r"
  Divide14/1 -> Trigonometric Function10/1
  Trigonometric Function10/1 -> Divide12/2
  Trigonometric Function11/1 -> Divide13/3
  Divide12/1 -> Trigonometric Function11/1

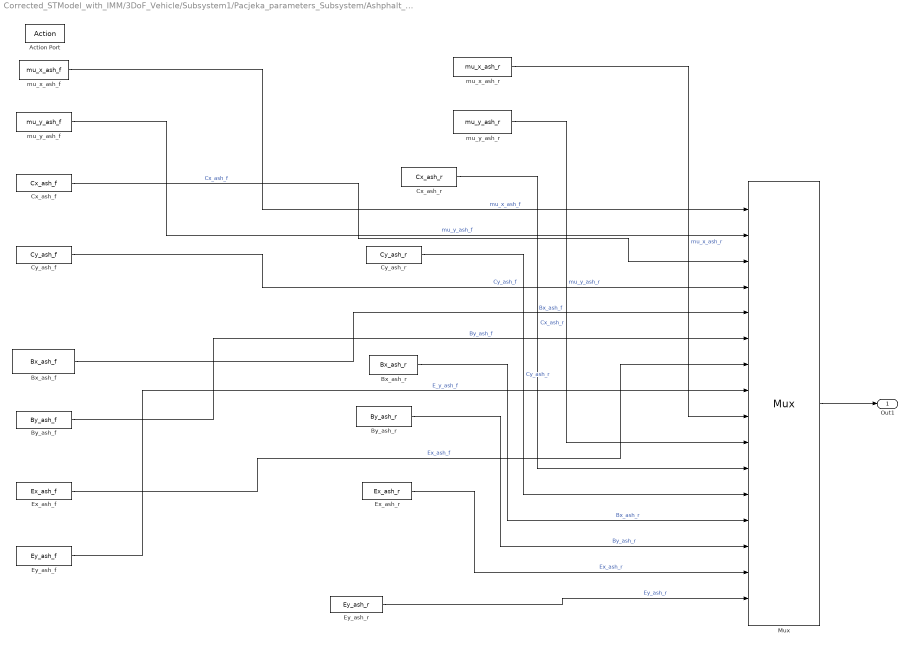
== system Corrected_STModel_with_IMM/3DoF_Vehicle/Subsystem1/Pacjeka_parameters_Subsystem/Ashphalt_condition_subsystem ==
  Action Port : ActionPort  ActionPortLabel=case [ 1 ]:
  Bx_ash_f : Constant  Value=Bx_ash_f
  Bx_ash_r : Constant  Value=Bx_ash_r
  By_ash_f : Constant  Value=By_ash_f
  By_ash_r : Constant  Value=By_ash_r
  Cx_ash_f : Constant  Value=Cx_ash_f
  Cx_ash_r : Constant  Value=Cx_ash_r
  Cy_ash_f : Constant  Value=Cy_ash_f
  Cy_ash_r : Constant  Value=Cy_ash_r
  Ex_ash_f : Constant  Value=Ex_ash_f
  Ex_ash_r : Constant  Value=Ex_ash_r
  Ey_ash_f : Constant  Value=Ey_ash_f
  Ey_ash_r : Constant  Value=Ey_ash_r
  Mux : Mux  Inputs=16
      settings: DisplayOption=signals
  mu_x_ash_f : Constant  Value=mu_x_ash_f
  mu_x_ash_r : Constant  Value=mu_x_ash_r
  mu_y_ash_f : Constant  Value=mu_y_ash_f
  mu_y_ash_r : Constant  Value=mu_y_ash_r
  Out1 : Outport  OutDataTypeStr=double  SampleTime=Ts  VectorParamsAs1DForOutWhenUnconnected=off
  wires:
  mu_x_ash_f/1 -> Mux/1  "mu_x_ash_f"
  mu_y_ash_f/1 -> Mux/2  "mu_y_ash_f"
  Cx_ash_f/1 -> Mux/3  "Cx_ash_f"
  Cy_ash_f/1 -> Mux/4  "Cy_ash_f"
  Bx_ash_f/1 -> Mux/5  "Bx_ash_f"
  By_ash_f/1 -> Mux/6  "By_ash_f"
  Ex_ash_f/1 -> Mux/7  "Ex_ash_f"
  Ey_ash_f/1 -> Mux/8  "E_y_ash_f"
  Cy_ash_r/1 -> Mux/12  "Cy_ash_r"
  Cx_ash_r/1 -> Mux/11  "Cx_ash_r"
  By_ash_r/1 -> Mux/14  "By_ash_r"
  Bx_ash_r/1 -> Mux/13  "Bx_ash_r"
  mu_y_ash_r/1 -> Mux/10  "mu_y_ash_r"
  Ex_ash_r/1 -> Mux/15  "Ex_ash_r"
  mu_x_ash_r/1 -> Mux/9  "mu_x_ash_r"
  Ey_ash_r/1 -> Mux/16  "Ey_ash_r"
  Mux/1 -> Out1/1

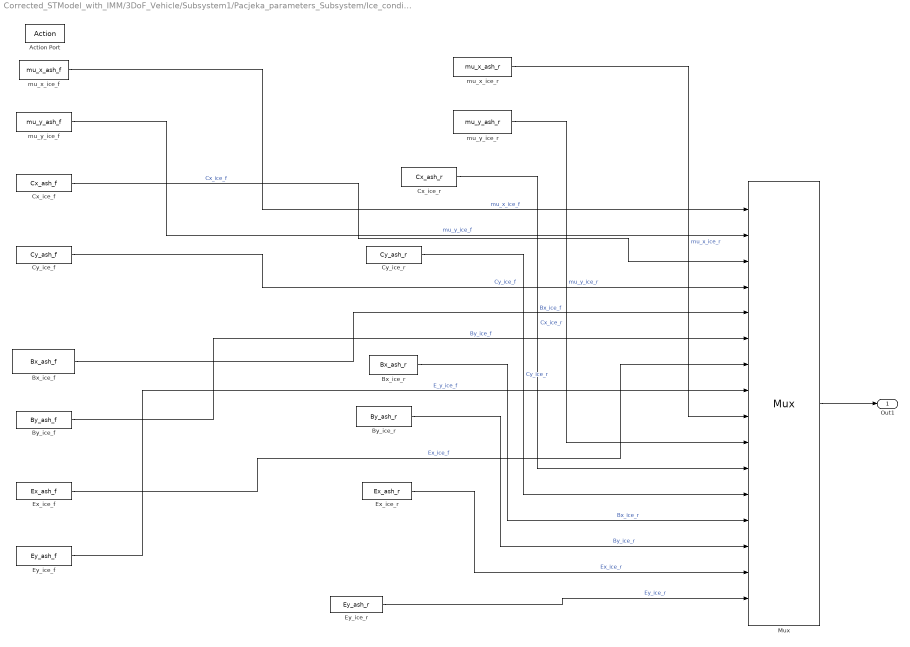
== system Corrected_STModel_with_IMM/3DoF_Vehicle/Subsystem1/Pacjeka_parameters_Subsystem/Ice_condition_subsystem ==
  Action Port : ActionPort  ActionPortLabel=case [ 4 ]:
  Bx_ice_f : Constant  Value=Bx_ash_f
  Bx_ice_r : Constant  Value=Bx_ash_r
  By_ice_f : Constant  Value=By_ash_f
  By_ice_r : Constant  Value=By_ash_r
  Cx_ice_f : Constant  Value=Cx_ash_f
  Cx_ice_r : Constant  Value=Cx_ash_r
  Cy_ice_f : Constant  Value=Cy_ash_f
  Cy_ice_r : Constant  Value=Cy_ash_r
  Ex_ice_f : Constant  Value=Ex_ash_f
  Ex_ice_r : Constant  Value=Ex_ash_r
  Ey_ice_f : Constant  Value=Ey_ash_f
  Ey_ice_r : Constant  Value=Ey_ash_r
  Mux : Mux  Inputs=16
      settings: DisplayOption=signals
  mu_x_ice_f : Constant  Value=mu_x_ash_f
  mu_x_ice_r : Constant  Value=mu_x_ash_r
  mu_y_ice_f : Constant  Value=mu_y_ash_f
  mu_y_ice_r : Constant  Value=mu_y_ash_r
  Out1 : Outport  OutDataTypeStr=double  SampleTime=Ts  VectorParamsAs1DForOutWhenUnconnected=off
  wires:
  mu_x_ice_f/1 -> Mux/1  "mu_x_ice_f"
  mu_y_ice_f/1 -> Mux/2  "mu_y_ice_f"
  Cx_ice_f/1 -> Mux/3  "Cx_ice_f"
  Cy_ice_f/1 -> Mux/4  "Cy_ice_f"
  Bx_ice_f/1 -> Mux/5  "Bx_ice_f"
  By_ice_f/1 -> Mux/6  "By_ice_f"
  Ex_ice_f/1 -> Mux/7  "Ex_ice_f"
  Ey_ice_f/1 -> Mux/8  "E_y_ice_f"
  Cy_ice_r/1 -> Mux/12  "Cy_ice_r"
  Cx_ice_r/1 -> Mux/11  "Cx_ice_r"
  By_ice_r/1 -> Mux/14  "By_ice_r"
  Bx_ice_r/1 -> Mux/13  "Bx_ice_r"
  mu_y_ice_r/1 -> Mux/10  "mu_y_ice_r"
  Ex_ice_r/1 -> Mux/15  "Ex_ice_r"
  mu_x_ice_r/1 -> Mux/9  "mu_x_ice_r"
  Ey_ice_r/1 -> Mux/16  "Ey_ice_r"
  Mux/1 -> Out1/1

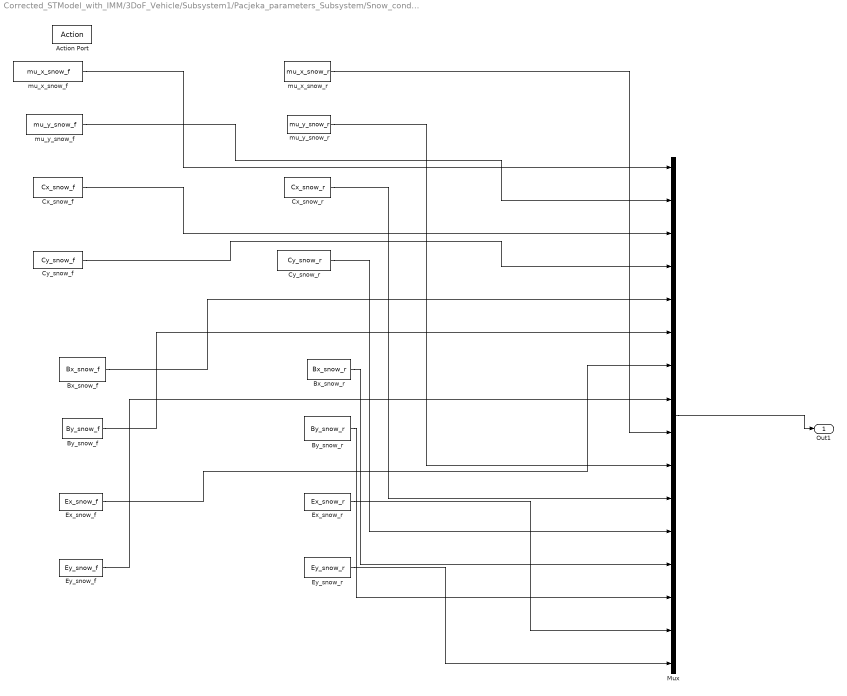
== system Corrected_STModel_with_IMM/3DoF_Vehicle/Subsystem1/Pacjeka_parameters_Subsystem/Snow_condition_subsystem ==
  Action Port : ActionPort  ActionPortLabel=case [ 3 ]:
  Bx_snow_f : Constant  Value=Bx_snow_f
  Bx_snow_r : Constant  Value=Bx_snow_r
  By_snow_f : Constant  Value=By_snow_f
  By_snow_r : Constant  Value=By_snow_r
  Cx_snow_f : Constant  Value=Cx_snow_f
  Cx_snow_r : Constant  Value=Cx_snow_r
  Cy_snow_f : Constant  Value=Cy_snow_f
  Cy_snow_r : Constant  Value=Cy_snow_r
  Ex_snow_f : Constant  Value=Ex_snow_f
  Ex_snow_r : Constant  Value=Ex_snow_r
  Ey_snow_f : Constant  Value=Ey_snow_f
  Ey_snow_r : Constant  Value=Ey_snow_r
  Mux : Mux  Inputs=16
  mu_x_snow_f : Constant  Value=mu_x_snow_f
  mu_x_snow_r : Constant  Value=mu_x_snow_r
  mu_y_snow_f : Constant  Value=mu_y_snow_f
  mu_y_snow_r : Constant  Value=mu_y_snow_r
  Out1 : Outport  OutDataTypeStr=double  SampleTime=Ts  VectorParamsAs1DForOutWhenUnconnected=off
  wires:
  Ex_snow_r/1 -> Mux/15
  Cy_snow_r/1 -> Mux/12
  By_snow_r/1 -> Mux/14
  Cx_snow_r/1 -> Mux/11
  mu_y_snow_r/1 -> Mux/10
  mu_x_snow_r/1 -> Mux/9
  Bx_snow_r/1 -> Mux/13
  Ey_snow_r/1 -> Mux/16
  mu_x_snow_f/1 -> Mux/1
  mu_y_snow_f/1 -> Mux/2
  Cx_snow_f/1 -> Mux/3
  Cy_snow_f/1 -> Mux/4
  Bx_snow_f/1 -> Mux/5
  By_snow_f/1 -> Mux/6
  Ex_snow_f/1 -> Mux/7
  Ey_snow_f/1 -> Mux/8
  Mux/1 -> Out1/1

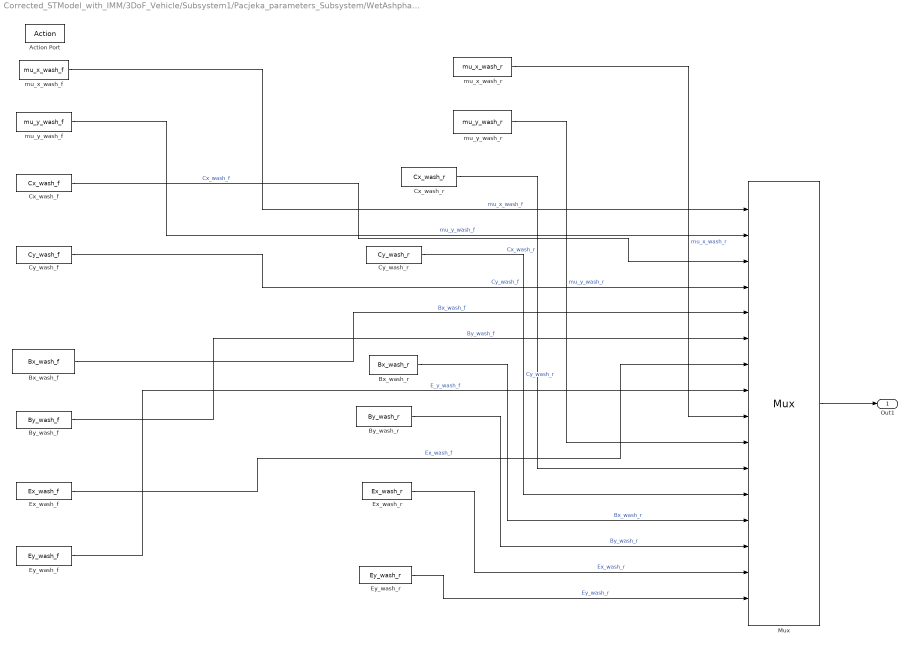
== system Corrected_STModel_with_IMM/3DoF_Vehicle/Subsystem1/Pacjeka_parameters_Subsystem/WetAshphalt_condition_subsystem ==
  Action Port : ActionPort  ActionPortLabel=case [ 2 ]:
  Bx_wash_f : Constant  Value=Bx_wash_f
  Bx_wash_r : Constant  Value=Bx_wash_r
  By_wash_f : Constant  Value=By_wash_f
  By_wash_r : Constant  Value=By_wash_r
  Cx_wash_f : Constant  Value=Cx_wash_f
  Cx_wash_r : Constant  Value=Cx_wash_r
  Cy_wash_f : Constant  Value=Cy_wash_f
  Cy_wash_r : Constant  Value=Cy_wash_r
  Ex_wash_f : Constant  Value=Ex_wash_f
  Ex_wash_r : Constant  Value=Ex_wash_r
  Ey_wash_f : Constant  Value=Ey_wash_f
  Ey_wash_r : Constant  Value=Ey_wash_r
  Mux : Mux  Inputs=16
      settings: DisplayOption=signals
  mu_x_wash_f : Constant  Value=mu_x_wash_f
  mu_x_wash_r : Constant  Value=mu_x_wash_r
  mu_y_wash_f : Constant  Value=mu_y_wash_f
  mu_y_wash_r : Constant  Value=mu_y_wash_r
  Out1 : Outport  OutDataTypeStr=double  SampleTime=Ts  VectorParamsAs1DForOutWhenUnconnected=off
  wires:
  mu_x_wash_f/1 -> Mux/1  "mu_x_wash_f"
  mu_y_wash_f/1 -> Mux/2  "mu_y_wash_f"
  Cx_wash_f/1 -> Mux/3  "Cx_wash_f"
  Cy_wash_f/1 -> Mux/4  "Cy_wash_f"
  Bx_wash_f/1 -> Mux/5  "Bx_wash_f"
  By_wash_f/1 -> Mux/6  "By_wash_f"
  Ex_wash_f/1 -> Mux/7  "Ex_wash_f"
  Ey_wash_f/1 -> Mux/8  "E_y_wash_f"
  Cy_wash_r/1 -> Mux/12  "Cy_wash_r"
  Cx_wash_r/1 -> Mux/11  "Cx_wash_r"
  By_wash_r/1 -> Mux/14  "By_wash_r"
  Bx_wash_r/1 -> Mux/13  "Bx_wash_r"
  mu_y_wash_r/1 -> Mux/10  "mu_y_wash_r"
  Ex_wash_r/1 -> Mux/15  "Ex_wash_r"
  mu_x_wash_r/1 -> Mux/9  "mu_x_wash_r"
  Ey_wash_r/1 -> Mux/16  "Ey_wash_r"
  Mux/1 -> Out1/1

== system Corrected_STModel_with_IMM/3DoF_Vehicle/Subsystem1/Vxdot_subsystem/Fy_subsystem ==
  Fyf : Inport
  Fxf : Inport  Port=2
  Fxr : Inport  Port=3
  cosDelta : Inport  Port=4
  sinDelta : Inport  Port=5
  Add : Sum
  Mux : Mux  Inputs=3
  Terminator : Terminator
  Fx : Outport  VectorParamsAs1DForOutWhenUnconnected=off
  wires:
  Add/1 -> Fx/1
  Fxf/1 -> Add/1
  Fxr/1 -> Add/2
  Mux/1 -> Terminator/1
  cosDelta/1 -> Mux/1
  sinDelta/1 -> Mux/2
  Fyf/1 -> Mux/3

== system Corrected_STModel_with_IMM/3DoF_Vehicle/Subsystem1/Vydot_subsystem/Fy_subsystem ==
  Fyf : Inport
  Fyr : Inport  Port=2
  Fxf : Inport  Port=3
  cosDelta : Inport  Port=4
  sinDelta : Inport  Port=5
  Add : Sum  Inputs=2
  Mux : Mux  Inputs=3
  Terminator : Terminator
  Fy : Outport  VectorParamsAs1DForOutWhenUnconnected=off
  wires:
  Add/1 -> Fy/1
  Fyf/1 -> Add/1
  Fyr/1 -> Add/2
  Fxf/1 -> Mux/1
  cosDelta/1 -> Mux/2
  sinDelta/1 -> Mux/3
  Mux/1 -> Terminator/1

== matlab function Corrected_STModel_with_IMM/MATLAB Function ==
  data: theta_sw_FH input; y output; T input
function y = fcn(theta_sw_FH,T)
    i=(T+0.001)/0.001;
    
y = theta_sw_FH(i);

== matlab function Corrected_STModel_with_IMM/Behavior Identification/MATLAB Function3 ==
  data: y_tilde input; u input; prenormalizedWts output; X input; P input; weights output; likelihood output; estimates output; comb_x output; comb_p output
function [prenormalizedWts, weights, likelihood, estimates, comb_x, comb_p]   = imm_laneChanges(y_tilde, u, X, P)
    persistent amm;
    
    if isempty(amm)
        Ts = 0.1;
        
        amm = HighwayScenarioIMMForVehD(Ts);
    end

    % mix initial states for the current cycle first
    amm.mixEstimates();

    % predict
    amm.predict(u);
    
    % correct and update probabilistic weights
    amm.correct(y_tilde);
    
    % combined estimates
    [comb_x, comb_p] = amm.calculateCombinedEstimate();
    
    prenormalizedWts = amm.getFilterNonNormalizedWeights();
    weights = amm.getFilterWeights();
    likelihood = amm.getFilterLikelihoods();
    estimates = amm.getFilterEstimates();
    
end
